simulink subsystem "fluids_and_control_subsystem_R2024a"  (R2024a)
settings: Solver=VariableStepAuto  StartTime=0.0  StopTime=10.0  RelTol=1e-3
undefined symbols (not defined in the file or in its folder): timestep
libraries: aircraft_refuel_control x1, simulink x1, GS_refuel_control x1
settings Model: Creator=MW  LastModifiedBy=MW

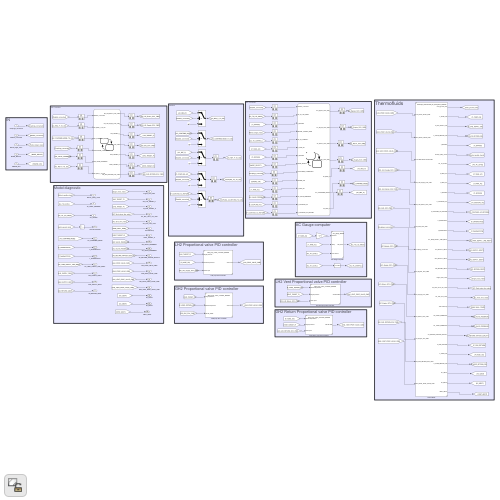
[thumbnail: Simulink's stored preview of the top-level diagram]
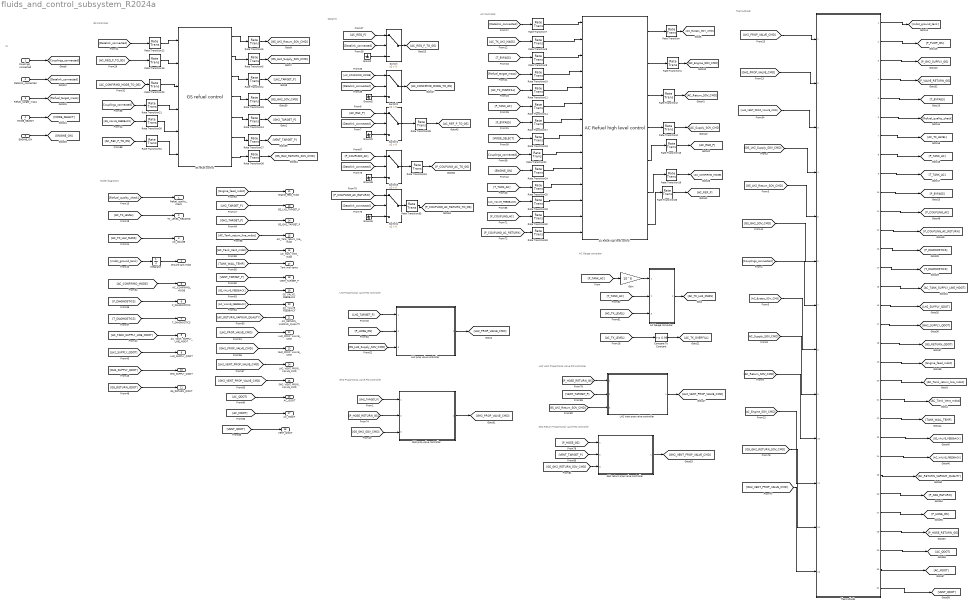
== system fluids_and_control_subsystem_R2024a ==
  note: AC Controller
  note: Model diagnostic
  note: LH2 Vent Proportional valve PID controller
  note: Thermofluids
  note: AC Gauge computer
  note: Datalink
  note: LH2 Proportional valve PID controller
  note: GH2 Proportional valve PID controller
  note: IN
  note: GS Controller
  note: GH2 Return Proportional valve PID controller
  Couplings_connected : Inport  OutDataTypeStr=boolean
  Datalink_connected : Inport  Port=2  OutDataTypeStr=boolean
  Refuel_target_mass : Inport  Port=3  OutDataTypeStr=double
  MODE_SELECT : Inport  Port=4  OutDataTypeStr=boolean
  ENGINE_ON : Inport  Port=5  OutDataTypeStr=boolean
  AC Gauge computer : Subsystem  ReferencedSubsystem=AC_gauge_R2024a
  AC Refuel high level control : aircraft_refuel_control/AC Refuel high level control  SystemSampleTime=timestep  VariantActivationTime=update diagram  AllowFlexibleInterface=on  Latency=0  AutoFrameSizeCalculation=off
  Compare To Constant : simulink/Logic and Bit Operations/Compare To Constant  relop=>=  const=0.99  OutDataTypeStr=boolean
  GH2 prop valve controller : Subsystem  ReferencedSubsystem=GH2_prop_valve_controller_R2024a
  GH2 return prop valve controller : Subsystem  ReferencedSubsystem=Vent_prop_valve_controller_R2024a
  GS refuel control : GS_refuel_control/GS refuel control  SystemSampleTime=timestep  VariantActivationTime=update diagram  AllowFlexibleInterface=on  Latency=0  AutoFrameSizeCalculation=off
  Gain : Gain  Gain=10^6
  Ground{,1..4} (5 alike) : Ground
  Integrator : Integrator
  LH2 Vent prop valve controller : Subsystem  ReferencedSubsystem=Vent_prop_valve_controller_R2024a
  LH2 prop valve controller : Subsystem  ReferencedSubsystem=LH2_prop_valve_controller_R2024a
  Rate Transition{,1..36} (37 alike) : RateTransition
  Switch : Switch  Criteria=u2 > Threshold  SaturateOnIntegerOverflow=off  InputSameDT=off
  Switch1 : Switch  Criteria=u2 > Threshold  OutDataTypeStr=double  SaturateOnIntegerOverflow=off  InputSameDT=off
  Switch2 : Switch  Criteria=u2 > Threshold  SaturateOnIntegerOverflow=off  InputSameDT=off
  Switch3 : Switch  Criteria=u2 > Threshold  OutDataTypeStr=double  SaturateOnIntegerOverflow=off  InputSameDT=off
  Switch4 : Switch  Criteria=u2 > Threshold  OutDataTypeStr=double  SaturateOnIntegerOverflow=off  InputSameDT=off
  Thermofluids : Subsystem  ReferencedSubsystem=simscape_thermofluids_full_subsystem_R2024a
  Refuel_quality_check : Outport
  TK_LEVEL_READING : Outport  Port=2
  AC_GAUGE : Outport  Port=3
  Ground tank Mdot : Outport  Port=4
  AC_CONFIRMD_MODE : Outport  Port=5
  P_DIAGNOSTICS : Outport  Port=6  OutDataTypeStr=Bus: P_DIAGNOSTIC
  T_DIAGNOSTICS : Outport  Port=7  OutDataTypeStr=Bus: T_DIAGNOSTIC
  AC_TANK_SUPPLY_LINE_MDOT : Outport  Port=8
  LH2_SUPPLY_QDOT : Outport  Port=9
  GH2_SUPPLY_QDOT : Outport  Port=10
  GS_RETURN_QDOT : Outport  Port=11
  Engine_feed_mdot : Outport  Port=12
  GS_LH2_TARGET_P : Outport  Port=13
  GS_GH2_TARGET_P : Outport  Port=14
  AC_Tank_return_line_mdot : Outport  Port=15
  AC_Tank_Vent_mdot : Outport  Port=16
  Tank wall temp : Outport  Port=17
  VENT_TARGET_P : Outport  Port=18
  GS_VALVE_FEEDBACK : Outport  Port=19  OutDataTypeStr=Bus: GS_VALVE_FEEDBACK
  AC_VALVE_FEEDBACK : Outport  Port=20  OutDataTypeStr=Bus: AC_VALVE_FEEDBACK
  AC_RETURN_VAPOUR_QUALITY : Outport  Port=21
  LH2_PROP_VALVE_CMD : Outport  Port=22
  GH2_PROP_VALVE_CMD : Outport  Port=23
  LH2_VENT_PROP_VALVE_CMD : Outport  Port=24
  GH2_VENT_PROP_VALVE_CMD : Outport  Port=25
  AC_QDOT : Outport  Port=26  OutDataTypeStr=Bus: AC_QDOT
  AC_MDOT : Outport  Port=27  OutDataTypeStr=Bus: AC_MDOT
  VENT_QDOT : Outport  Port=28  OutDataTypeStr=Bus: VENT_QDOT
  wires:
  [GH2_PROP_VALVE_CMD] -> Thermofluids/2
  [GS_LH2_Return_SOV_CMD] -> Thermofluids/5
  [LH2_VENT_PROP_VALVE_CMD] -> Thermofluids/3
  Thermofluids/22 -> [TANK_WALL_TEMP]
  Thermofluids/23 -> [GS_VALVE_FEEDBACK]
  Thermofluids/19 -> [Engine_feed_mdot]
  Thermofluids/20 -> [AC_Tank_return_line_mdot]
  Thermofluids/14 -> [T_DIAGNOSTICS]
  Thermofluids/10 -> [P_BYPASS]
  Thermofluids/18 -> [GS_RETURN_QDOT]
  Thermofluids/21 -> [AC_Tank_Vent_mdot]
  Thermofluids/12 -> [P_COUPLING_AC_RETURN]
  Thermofluids/5 -> [T_BYPASS]
  Thermofluids/7 -> [AC_TK_LEVEL]
  Thermofluids/3 -> [P_GH2_SUPPLY_GS]
  Thermofluids/16 -> [LH2_SUPPLY_QDOT]
  Thermofluids/15 -> [AC_TANK_SUPPLY_LINE_MDOT]
  Thermofluids/8 -> [P_TANK_AC]
  Thermofluids/17 -> [GH2_SUPPLY_QDOT]
  Thermofluids/9 -> [T_TANK_AC]
  Thermofluids/2 -> [P_PUMP_GS]
  Thermofluids/6 -> [Refuel_quality_check]
  [AC_Return_SOV_CMD] -> Thermofluids/10
  [AC_Engine_SOV_CMD] -> Thermofluids/11
  AC Refuel high level control/3 -> Rate Transition2/1
  Rate Transition21/1 -> GS refuel control/4
  Compare To Constant/1 -> [AC_TK_OVERFILL]
  [T_TANK_AC] -> Rate Transition25/1
  Ground1/1 -> Switch1/3
  Thermofluids/4 -> [P_VALVE_RETURN_GS]
  [GH2_TARGET_P] -> GH2 prop valve controller/1
  [GH2_SUPPLY_QDOT] -> GH2_SUPPLY_QDOT/1
  Rate Transition10/1 -> AC Refuel high level control/4
  Rate Transition34/1 -> [P_COUPLING_AC_TO_GS]
  ENGINE_ON/1 -> [ENGINE_ON]
  GS refuel control/5 -> Rate Transition13/1
  [Datalink_connected] -> Switch3/2
  Thermofluids/24 -> [AC_VALVE_FEEDBACK]
  Rate Transition25/1 -> AC Refuel high level control/11
  Integrator/1 -> Ground tank Mdot/1
  Rate Transition/1 -> [AC_Bypass_SOV_CMD]
  Rate Transition5/1 -> [GS_LH2_Supply_SOV_CMD]
  [AC_REF_P_TO_GS] -> Rate Transition31/1
  LH2 Vent prop valve controller/1 -> [LH2_VENT_PROP_VALVE_CMD]
  [AC_VALVE_FEEDBACK] -> AC_VALVE_FEEDBACK/1
  Rate Transition7/1 -> AC Refuel high level control/1
  [P_COUPLING_AC] -> Rate Transition32/1
  Rate Transition14/1 -> AC Refuel high level control/6
  [AC_CONFIRMD_MODE] -> Switch2/1
  [LH2_SUPPLY_QDOT] -> LH2_SUPPLY_QDOT/1
  [AC_CONFIRMD_MODE] -> AC_CONFIRMD_MODE/1
  GS refuel control/6 -> Rate Transition27/1
  [VENT_TARGET_P] -> LH2 Vent prop valve controller/2
  Ground2/1 -> Switch2/3
  [AC_REQ_P_TO_GS] -> Rate Transition16/1
  Rate Transition26/1 -> [AC_REF_P]
  Ground3/1 -> Switch3/3
  [T_DIAGNOSTICS] -> T_DIAGNOSTICS/1
  AC Refuel high level control/6 -> Rate Transition19/1
  [AC_TK_LEVEL] -> AC Gauge computer/3
  Rate Transition19/1 -> [AC_CONFIRMD_MODE]
  [ENGINE_ON] -> Rate Transition24/1
  Ground/1 -> Switch/3
  AC Refuel high level control/4 -> Rate Transition3/1
  [AC_TK_OVERFILL] -> Rate Transition11/1
  [Datalink_connected] -> Rate Transition7/1
  [GS_GH2_SOV_CMD] -> GH2 prop valve controller/3
  [AC_TK_LH2_MASS] -> Rate Transition8/1
  GS refuel control/2 -> Rate Transition5/1
  [Engine_feed_mdot] -> Engine_feed_mdot/1
  Rate Transition27/1 -> [VENT_TARGET_P]
  [AC_Tank_Vent_mdot] -> AC_Tank_Vent_mdot/1
  [GS_VALVE_FEEDBACK] -> GS_VALVE_FEEDBACK/1
  Rate Transition30/1 -> GS refuel control/5
  Switch2/1 -> [AC_CONFIRMD_MODE_TO_GS]
  [MODE_SELECT] -> Rate Transition18/1
  [GS_RETURN_QDOT] -> GS_RETURN_QDOT/1
  [AC_VALVE_FEEDBACK] -> Rate Transition29/1
  Switch3/1 -> Rate Transition34/1
  Datalink_connected/1 -> [Datalink_connected]
  Switch/1 -> [AC_REQ_P_TO_GS]
  AC Refuel high level control/5 -> Rate Transition15/1
  [Couplings_connected] -> Rate Transition21/1
  [P_COUPLING_AC_RETURN] -> Switch4/1
  AC Refuel high level control/2 -> Rate Transition1/1
  [LH2_TARGET_P] -> GS_LH2_TARGET_P/1
  Rate Transition22/1 -> AC Refuel high level control/9
  Thermofluids/11 -> [P_COUPLING_AC]
  Rate Transition9/1 -> AC Refuel high level control/3
  [Refuel_quality_check] -> Refuel_quality_check/1
  Rate Transition6/1 -> [GS_LH2_Return_SOV_CMD]
  LH2 prop valve controller/1 -> [LH2_PROP_VALVE_CMD]
  [Datalink_connected] -> Switch1/2
  [P_TANK_AC] -> Rate Transition14/1
  Rate Transition35/1 -> [P_COUPLING_AC_RETURN_TO_GS]
  Rate Transition11/1 -> AC Refuel high level control/5
  [P_DIAGNOSTICS] -> P_DIAGNOSTICS/1
  Rate Transition4/1 -> [LH2_TARGET_P]
  Rate Transition33/1 -> AC Refuel high level control/14
  Rate Transition32/1 -> AC Refuel high level control/13
  AC Refuel high level control/7 -> Rate Transition26/1
  Gain/1 -> AC Gauge computer/1
  Rate Transition17/1 -> AC Refuel high level control/7
  [P_HOSE_RETURN_GS] -> GH2 prop valve controller/2
  [Datalink_connected] -> Switch2/2
  AC Refuel high level control/1 -> Rate Transition/1
  [GS_LH2_Supply_SOV_CMD] -> Thermofluids/4
  [AC_TK_LEVEL] -> TK_LEVEL_READING/1
  [Datalink_connected] -> Rate Transition12/1
  GH2 prop valve controller/1 -> [GH2_PROP_VALVE_CMD]
  [P_HOSE_GS] -> LH2 prop valve controller/2
  [LH2_PROP_VALVE_CMD] -> Thermofluids/1
  [T_TANK_AC] -> AC Gauge computer/2
  [GH2_TARGET_P] -> GS_GH2_TARGET_P/1
  [GS_VALVE_FEEDBACK] -> Rate Transition30/1
  [AC_TK_LEVEL] -> Compare To Constant/1
  Thermofluids/1 -> [mdot_ground_tank]
  Rate Transition18/1 -> AC Refuel high level control/8
  [Datalink_connected] -> Switch4/2
  Switch1/1 -> Rate Transition28/1
  MODE_SELECT/1 -> [MODE_SELECT]
  [VENT_TARGET_P] -> VENT_TARGET_P/1
  Rate Transition2/1 -> [AC_Return_SOV_CMD]
  Switch4/1 -> Rate Transition35/1
  [TANK_WALL_TEMP] -> Tank wall temp/1
  [AC_CONFIRMD_MODE_TO_GS] -> Rate Transition20/1
  [AC_REF_P] -> Switch1/1
  [AC_TK_LH2_MASS] -> AC_GAUGE/1
  AC Gauge computer/1 -> [AC_TK_LH2_MASS]
  [Refuel_target_mass] -> Rate Transition10/1
  Rate Transition29/1 -> AC Refuel high level control/12
  Rate Transition16/1 -> GS refuel control/2
  [AC_Supply_SOV_CMD] -> Thermofluids/9
  Couplings_connected/1 -> [Couplings_connected]
  Rate Transition28/1 -> [AC_REF_P_TO_GS]
  [AC_Tank_return_line_mdot] -> AC_Tank_return_line_mdot/1
  Rate Transition31/1 -> GS refuel control/6
  Rate Transition24/1 -> AC Refuel high level control/10
  GS refuel control/1 -> Rate Transition6/1
  Rate Transition3/1 -> [AC_Supply_SOV_CMD]
  Rate Transition1/1 -> [AC_Engine_SOV_CMD]
  GS refuel control/4 -> Rate Transition23/1
  [T_BYPASS] -> Rate Transition9/1
  [P_HOSE_RETURN_GS] -> LH2 Vent prop valve controller/1
  [LH2_TARGET_P] -> LH2 prop valve controller/1
  [AC_TANK_SUPPLY_LINE_MDOT] -> AC_TANK_SUPPLY_LINE_MDOT/1
  Refuel_target_mass/1 -> [Refuel_target_mass]
  [mdot_ground_tank] -> Integrator/1
  Rate Transition15/1 -> [AC_REQ_P]
  [P_BYPASS] -> Rate Transition17/1
  Rate Transition12/1 -> GS refuel control/1
  Ground4/1 -> Switch4/3
  Rate Transition23/1 -> [GS_GH2_SOV_CMD]
  Rate Transition8/1 -> AC Refuel high level control/2
  [Datalink_connected] -> Switch/2
  Rate Transition20/1 -> GS refuel control/3
  [Couplings_connected] -> Thermofluids/7
  [P_COUPLING_AC] -> Switch3/1
  [P_COUPLING_AC_RETURN] -> Rate Transition33/1
  GS refuel control/3 -> Rate Transition4/1
  [GS_LH2_Supply_SOV_CMD] -> LH2 prop valve controller/3
  [Couplings_connected] -> Rate Transition22/1
  [P_TANK_AC] -> Gain/1
  [AC_Bypass_SOV_CMD] -> Thermofluids/8
  Thermofluids/13 -> [P_DIAGNOSTICS]
  [AC_REQ_P] -> Switch/1
  Rate Transition13/1 -> [GH2_TARGET_P]
  [GS_GH2_SOV_CMD] -> Thermofluids/6
  Thermofluids/25 -> [AC_RETURN_VAPOUR_QUALITY]
  [AC_RETURN_VAPOUR_QUALITY] -> AC_RETURN_VAPOUR_QUALITY/1
  [LH2_PROP_VALVE_CMD] -> LH2_PROP_VALVE_CMD/1
  [GH2_PROP_VALVE_CMD] -> GH2_PROP_VALVE_CMD/1
  [LH2_VENT_PROP_VALVE_CMD] -> LH2_VENT_PROP_VALVE_CMD/1
  GH2 return prop valve controller/1 -> [GH2_VENT_PROP_VALVE_CMD]
  [P_HOSE_GS] -> GH2 return prop valve controller/1
  [VENT_TARGET_P] -> GH2 return prop valve controller/2
  [GH2_VENT_PROP_VALVE_CMD] -> Thermofluids/13
  Rate Transition36/1 -> [GS_GH2_RETURN_SOV_CMD]
  GS refuel control/7 -> Rate Transition36/1
  [GS_GH2_RETURN_SOV_CMD] -> Thermofluids/12
  Thermofluids/26 -> [P_GAS_RETURN]
  [GS_GH2_RETURN_SOV_CMD] -> GH2 return prop valve controller/3
  [GS_LH2_Return_SOV_CMD] -> LH2 Vent prop valve controller/3
  [GH2_VENT_PROP_VALVE_CMD] -> GH2_VENT_PROP_VALVE_CMD/1
  Thermofluids/28 -> [P_HOSE_RETURN_GS]
  Thermofluids/27 -> [P_HOSE_GS]
  [AC_QDOT] -> AC_QDOT/1
  Thermofluids/29 -> [AC_QDOT]
  Thermofluids/30 -> [AC_MDOT]
  [AC_MDOT] -> AC_MDOT/1
  [VENT_QDOT] -> VENT_QDOT/1
  Thermofluids/31 -> [VENT_QDOT]
